simulink model "MPC_implemented_wout_constr"  (R2023b)
settings: Solver=VariableStepAuto  StartTime=0.0  StopTime=30  RelTol=1e-3
StartFcn:
  | ts = 1e-2;
  | 
  | feedin = 1;
  | feedout = [1 2];
  | F_s = feedback(lin_sys_ss,K_s,feedin,feedout,-1);
  | F_s = minreal(F_s);
  | 
  | F_k = c2d(F_s,ts);
  | 
  | Fk_A = F_k.A;
  | Fk_B1 = F_k.B(:,1);
  | Fk_C = F_k.C;
values from neighbouring files (symbols this model uses):
  Gamma = CZ*Gamma    [constr_matrix.m]    (also in mpc_without_constr.m)
  Kmpc = Kfull(1,:)    [mpc_without_constr.m]
  Psi = CZ*Psi    [constr_matrix.m]    (also in mpc_without_constr.m)
  T = zeros(l*Hp,m)    [constr_matrix.m]    (also in mpc_without_constr.m)
undefined symbols (not defined in the file or in its folder): DiscIntNeverNeededParam, dist, Xi
libraries: cstblocks x2, dspsrcs4 x2
settings Model: Creator=aniello  LastModifiedBy=aniello
settings DebuggingCC: UnderSpecifiedDimensionMsg=warning

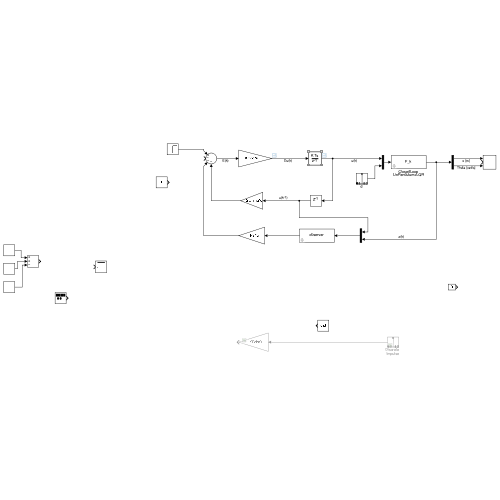
[thumbnail: Simulink's stored preview of the top-level diagram]
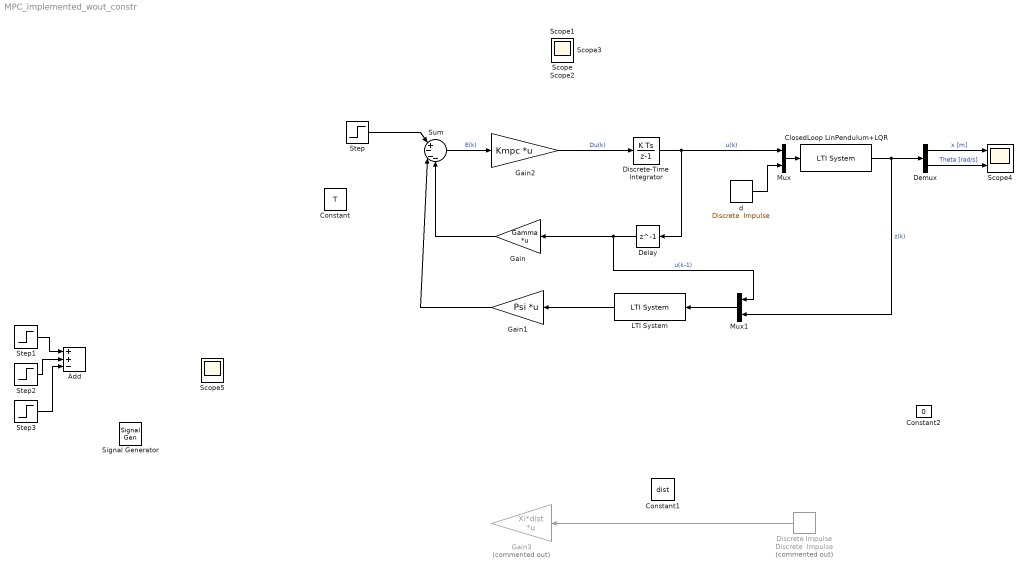
== system MPC_implemented_wout_constr ==
  Add : Sum  Inputs=++-
  ClosedLoop LinPendulum+LQR : cstblocks/LTI System  sys=F_k  IC=[]  PadeOrder=0
  Constant : Constant  Value=T
  Constant1 : Constant  Value=dist
  Constant2 : Constant  Value=0
  Delay : Delay  DelayLength=1  SampleTime=ts
  Demux : Demux  Outputs=2
  Discrete Impulse : dspsrcs4/Discrete  Impulse  Commented=on  Delay=800  SampleTime=0.02  FrameSample=1  OutputFrames=off  dataType=double  isSigned=on  wordLen=16  udDataType=sfix(16)  fracBitsMode=Best precision  numFracBits=15  OutDataTypeStr=double  LastOutDataTypeStr=double
  Discrete-Time Integrator : DiscreteIntegrator  SampleTime=ts  ICPrevOutput=DiscIntNeverNeededParam  ICPrevScaledInput=DiscIntNeverNeededParam
  Gain : Gain  Gain=Gamma  Multiplication=Matrix(K*u)
  Gain1 : Gain  Gain=Psi  Multiplication=Matrix(K*u)
  Gain2 : Gain  Gain=Kmpc  Multiplication=Matrix(K*u)
  Gain3 : Gain  Commented=on  Gain=Xi*dist  Multiplication=Matrix(K*u)
  LTI System : cstblocks/LTI System  sys=observer  IC=[]  PadeOrder=0
  Mux : Mux  Inputs=2
  Mux1 : Mux  Inputs=2
  Scope4 : Scope  NumInputPorts=3
  Scope{,1..3,5} (5 alike) : Scope
  Signal Generator : SignalGenerator  Frequency=0.3  Units=rad/sec
  Step : Step  Time=0  SampleTime=0
  Step1 : Step  SampleTime=0
  Step2 : Step  Time=8  After=2  SampleTime=0
  Step3 : Step  Time=15  After=3  SampleTime=0
  Sum : Sum  Inputs=|+---
  d : dspsrcs4/Discrete  Impulse  Delay=800  SampleTime=0.02  FrameSample=1  OutputFrames=off  dataType=double  isSigned=on  wordLen=16  udDataType=sfix(16)  fracBitsMode=Best precision  numFracBits=15  OutDataTypeStr=double  LastOutDataTypeStr=double
  wires:
  Mux/1 -> ClosedLoop LinPendulum+LQR/1
  Mux1/1 -> LTI System/1
  Discrete-Time Integrator/1 -> Mux/1, Delay/1  "u(k)"
  ClosedLoop LinPendulum+LQR/1 -> Mux1/2, Demux/1  "z(k)"
  Delay/1 -> Mux1/1, Gain/1  "u(k-1)"
  LTI System/1 -> Gain1/1
  Gain2/1 -> Discrete-Time Integrator/1  "Du(k)"
  Sum/1 -> Gain2/1  "E(k)"
  Demux/1 -> Scope4/1  "x [m]"
  Demux/2 -> Scope4/3  "Theta [rad/s]"
  Step1/1 -> Add/1
  Step2/1 -> Add/2
  Step3/1 -> Add/3
  Gain/1 -> Sum/4
  Gain1/1 -> Sum/3
  Step/1 -> Sum/1
  Discrete Impulse/1 -> Gain3/1
  d/1 -> Mux/2
